simulink model "TRDP_head_verify"  (R2021a)
settings: configuration reference "ART_1G_IDS_Speedgoat" (kept outside this file)
libraries: commutil2 x20, etargetslib x2, simulink x1
settings Model: DataDictionary=Model_Config.sldd  Creator=xinrui  LastModifiedBy=xinrui
settings ConfigSetRef: SourceName=ART_1G_IDS_Speedgoat

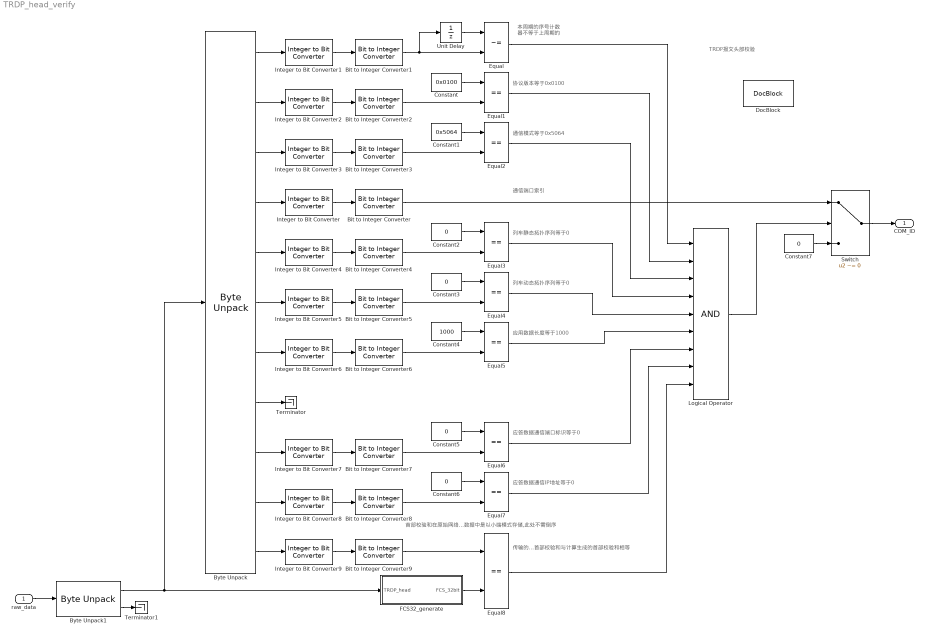
== system TRDP_head_verify ==
  note: 本周期的序号计数
      | 器不等于上周期的
  note: 协议版本等于0x0100
  note: 通信模式等于0x5064
  note: 列车静态拓扑序列等于0
  note: 列车动态拓扑序列等于0
  note: 应用数据长度等于1000
  note: 应答数据通信端口标识等于0
  note: 应答数据通信IP地址等于0
  note: 首部校验和在原始网络数据中是以小端模式存储,此处不需倒序
  note: 传输的首部校验和与计算生成的首部校验和相等
  note: 通信端口索引
  note: TRDP报文头部校验
  raw_data : Inport  OutDataTypeStr=uint8  PortDimensions=1040
  Bit to Integer Converter{,1,4..8} (7 alike) : commutil2/Bit to Integer Converter  nbits=32  bitOrder=MSB first  signedOutputValues=Unsigned  outDtype=uint32  outDtypeSigned=Inherit via internal rule
  Bit to Integer Converter2 : commutil2/Bit to Integer Converter  nbits=16  bitOrder=MSB first  signedOutputValues=Unsigned  outDtype=uint16  outDtypeSigned=Inherit via internal rule
  Bit to Integer Converter3 : commutil2/Bit to Integer Converter  nbits=16  bitOrder=MSB first  signedOutputValues=Unsigned  outDtype=uint16  outDtypeSigned=Inherit via internal rule
  Bit to Integer Converter9 : commutil2/Bit to Integer Converter  nbits=32  bitOrder=LSB first  signedOutputValues=Unsigned  outDtype=uint32  outDtypeSigned=Inherit via internal rule
  Byte Unpack : etargetslib/Byte Unpack  dimensions={[4],[2],[2],[4],[4],[4],[4],[4],[4],[4],[4]}  datatypes={'uint8','uint8','uint8','uint8','uint8','uint8','uint8','uint8','uint8','uint8','uint8'}  byteAlign=1
  Byte Unpack1 : etargetslib/Byte Unpack  dimensions={[40],[1000]}  datatypes={'uint8','uint8'}  byteAlign=1
  Constant : Constant  Value=0x0100  OutDataTypeStr=uint16  SampleTime=-1
  Constant1 : Constant  Value=0x5064  OutDataTypeStr=uint16  SampleTime=-1
  Constant{2..3,5..7} (5 alike) : Constant  Value=0  OutDataTypeStr=uint32  SampleTime=-1
  Constant4 : Constant  Value=1000  OutDataTypeStr=uint32  SampleTime=-1
  DocBlock : simulink/Model-Wide Utilities/DocBlock  DocumentType=HTML  mask(DocBlock){}
      mask Display:
      | plot([.8 0 0 1 1 .8 .8 1],[1 1 0 0 .8 1 .8 .8]);
      | text(.5,.6,'CHANGELOG','horizontalalignment','center');
      | text(.95,.05,get_param(gcb,'DocumentType'),'verticalalignment','bottom','horizontalalignment','right');
  Equal : RelationalOperator  Operator=~=  OutDataTypeStr=boolean  RndMeth=Simplest
  Equal{1..8} (8 alike) : RelationalOperator  Operator===  OutDataTypeStr=boolean  RndMeth=Simplest
  FCS32_generate : MATLAB Function  TreatAsAtomicUnit=on
  Integer to Bit Converter{,1..8} (9 alike) : commutil2/Integer to Bit Converter  nbits=8  signedInputValues=Unsigned  bitOrder=MSB first  outDtype=Inherit via internal rule
  Integer to Bit Converter9 : commutil2/Integer to Bit Converter  nbits=8  signedInputValues=Unsigned  bitOrder=LSB first  outDtype=Inherit via internal rule
  Logical Operator : Logic  Inputs=9  AllPortsSameDT=off  OutDataTypeStr=boolean
  Switch : Switch  Criteria=u2 ~= 0
  Terminator : Terminator
  Terminator1 : Terminator
  Unit Delay : UnitDelay  SampleTime=-1  HasFrameUpgradeWarning=on
  COM_ID : Outport  OutDataTypeStr=uint32  PortDimensions=1
  wires:
  Switch/1 -> COM_ID/1
  Integer to Bit Converter/1 -> Bit to Integer Converter/1
  Unit Delay/1 -> Equal/1
  Byte Unpack/4 -> Integer to Bit Converter/1
  Constant/1 -> Equal1/1
  Constant1/1 -> Equal2/1
  Constant2/1 -> Equal3/1
  Integer to Bit Converter1/1 -> Bit to Integer Converter1/1
  Bit to Integer Converter1/1 -> Equal/2, Unit Delay/1
  Byte Unpack/1 -> Integer to Bit Converter1/1
  Integer to Bit Converter2/1 -> Bit to Integer Converter2/1
  Byte Unpack/2 -> Integer to Bit Converter2/1
  Bit to Integer Converter2/1 -> Equal1/2
  Integer to Bit Converter3/1 -> Bit to Integer Converter3/1
  Byte Unpack/3 -> Integer to Bit Converter3/1
  Bit to Integer Converter3/1 -> Equal2/2
  Integer to Bit Converter4/1 -> Bit to Integer Converter4/1
  Byte Unpack/5 -> Integer to Bit Converter4/1
  Bit to Integer Converter4/1 -> Equal3/2
  Bit to Integer Converter5/1 -> Equal4/2
  Integer to Bit Converter5/1 -> Bit to Integer Converter5/1
  Constant3/1 -> Equal4/1
  Byte Unpack/6 -> Integer to Bit Converter5/1
  Constant4/1 -> Equal5/1
  Integer to Bit Converter6/1 -> Bit to Integer Converter6/1
  Bit to Integer Converter6/1 -> Equal5/2
  Byte Unpack/7 -> Integer to Bit Converter6/1
  Byte Unpack/8 -> Terminator/1
  Constant5/1 -> Equal6/1
  Integer to Bit Converter7/1 -> Bit to Integer Converter7/1
  Bit to Integer Converter7/1 -> Equal6/2
  Byte Unpack/9 -> Integer to Bit Converter7/1
  Bit to Integer Converter8/1 -> Equal7/2
  Integer to Bit Converter8/1 -> Bit to Integer Converter8/1
  Constant6/1 -> Equal7/1
  Byte Unpack/10 -> Integer to Bit Converter8/1
  Integer to Bit Converter9/1 -> Bit to Integer Converter9/1
  Byte Unpack/11 -> Integer to Bit Converter9/1
  raw_data/1 -> Byte Unpack1/1
  Byte Unpack1/2 -> Terminator1/1
  Byte Unpack1/1 -> Byte Unpack/1, FCS32_generate/1(TRDP_head)
  Bit to Integer Converter9/1 -> Equal8/1
  FCS32_generate/1(FCS_32bit) -> Equal8/2
  Constant7/1 -> Switch/3
  Equal8/1 -> Logical Operator/9
  Equal7/1 -> Logical Operator/8
  Equal6/1 -> Logical Operator/7
  Equal5/1 -> Logical Operator/6
  Equal4/1 -> Logical Operator/5
  Equal3/1 -> Logical Operator/4
  Equal2/1 -> Logical Operator/3
  Equal1/1 -> Logical Operator/2
  Equal/1 -> Logical Operator/1
  Logical Operator/1 -> Switch/2
  Bit to Integer Converter/1 -> Switch/1

== matlab function TRDP_head_verify/FCS32_generate ==
  data: TRDP_head input uint8 size=40; FCS_32bit output uint32 size=1
% 首部校验和生成
function FCS_32bit = FCS32_generate(TRDP_head)
%   1.输入参数：
%       (1)TRDP_head    TRDP头部数据
%   2.输出参数：
%       (1)FCS_32bit    计算生成的首部校验和

% 调用计算公式求解首部校验和，参与计算的原始数据为TRDP头部数据前36个字节
FCS_32bit = FCS32_calculate(TRDP_head, 36);

end
